simulink model "Function_Approximation_Ex1"  (R2024a)
settings: Solver=VariableStepAuto  StartTime=0.0  StopTime=512  RelTol=1e-3
undefined symbols (not defined in the file): S, vsva2197, xcvc1902
libraries: aieDSP x1, aieUtilities x1, vmcUtilities x1
settings Model: Creator=raghug  LastModifiedBy=sdegala
settings ConfigComp: CovBoundaryAbsTol=1.0e-5

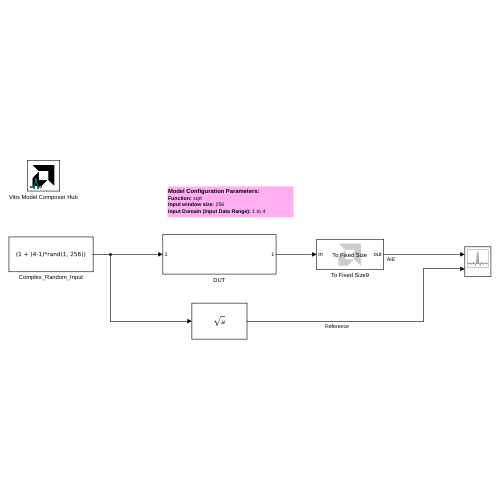
[thumbnail: Simulink's stored preview of the top-level diagram]
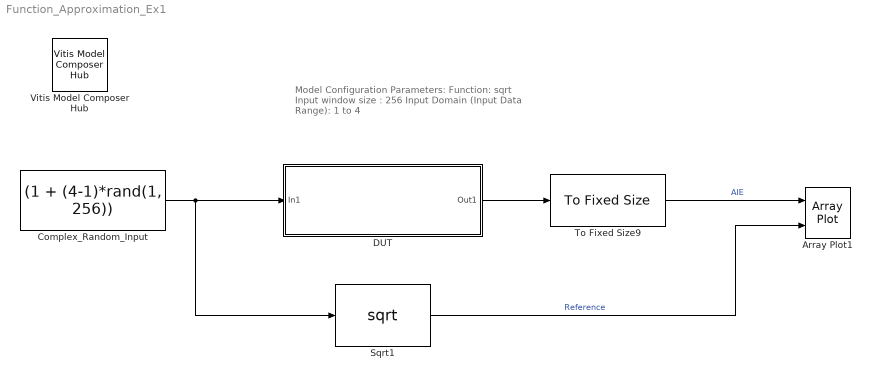
== system Function_Approximation_Ex1 ==
  note: Model Configuration Parameters:
      | Function: sqrt
      | Input window size : 256
      | Input Domain (Input Data Range): 1 to 4
  Array Plot1 : ArrayPlot  NumInputPorts=2  WindowPosition=[863.000000,486.000000,800.000000,500.000000,]  Visible=on  ScopeFrameLocation=window  YLimits=[0.8802 2.1161]  ShowLegend=on
  Complex_Random_Input : Constant  Value=(1 + (4-1)*rand(1, 256))  OutDataTypeStr=single  SampleTime=1
  DUT : Subsystem
  Sqrt1 : Sqrt
  To Fixed Size9 : aieUtilities/To Fixed Size  Mode=Stop simulation when input variable-size signal is not full  OutputSize=Inherit: Same as input  CopyMethod=Buffer samples to form output  HasStatusOutput=on
  Vitis Model Composer Hub : vmcUtilities/Vitis Model Composer Hub  Tag=genX  CodeGeneration=off  StartColumn=1  NumberOfColumns=1  TargetDirectory=./code  exportDesign=off  analyzeDesign=off  validateDesignOnHw=off  ExportType=AI Engines  IpVendor=xilinx.com  IpLibrary=hls  IpVersion=1.0  IpHWLanguage=Verilog  AieCompilerOptions={}  AieSimulatorOptions={}  CreateTestbench=off  TestbenchStackSize=10  RunRtlSim=off  RunCSim=off  RunAieSim=off  AieSimTimeout=50000  RunAieSimProfiling=off  LaunchVitisAnalyzer=off  PlotOutput=off  RunX86Sim=off  X86SimTimeout=10  GenHwImage=off  GenLibadfXo=off  GenHwValidationCode=off  PlatformType=Not Specified  HwSystemType=Baremetal  HwValidationTarget=hw  ProjDevice=xcvc1902-vsva2197-1LP-e-S  ProjDevicePart=xcvc1902-vsva2197-1LP-e-S  AIEType=AIE  SamplePeriod=-1  ClockFrequency=200  DataPathParallelism=1  xilinxfamily=versalaicore  part=xcvc1902  speed=-1LP-e-S  package=vsva2197  directory=./netlist  testbench=off  incr_netlist=off  synthesis_tool=Vivado  clock_wrapper=Clock Enables  dbl_ovrd=According to Block Masks  dcm_input_clock_period=10  sysclk_period=10  simulink_period=1  eval_field=0  LogFileName=''  NThreads=4
  wires:
  Complex_Random_Input/1 -> DUT/1(In1), Sqrt1/1
  To Fixed Size9/1 -> Array Plot1/1  "AIE"
  Sqrt1/1 -> Array Plot1/2  "Reference"
  DUT/1(Out1) -> To Fixed Size9/1

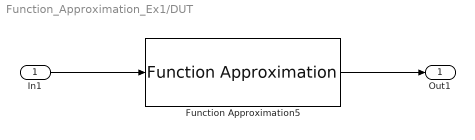
== system Function_Approximation_Ex1/DUT ==
  In1 : Inport
  Function Approximation5 : aieDSP/Function Approximation  AIE_VARIANT=1  data_type=float  coarse_bits=8  fine_bits=7  domain_mode=1 to 4 (2)  num_frames=256  shift_output=0  rnd_mode=Floor  sat_mode=Saturate  use_lut_reload=off  lookup_values=sqrt  blockJsonConstraints=[]  blockJsonConstraintsInternal=[]  spec=vmc_func_approx.json  SerializedMaskParamNames=[]  SerializedMaskParamValues=[]  SerializedMaskParamVisibilities=[]  block_type=Function Approximation  SerializedMaskParamDataypes=uint|typename|uint|uint|uint|uint|uint|uint|uint|uint|data_type  SerializedMaskParamEnumStrArr=0|0|0|0|0 to 1 (0),1 to 2 (1),1 to 4 (2)|0|0|Floor,Ceiling,Round to positive infinity,Round to negative infinity,Round symmetrical to infinity,Round symmetrical to zero,Round convergent to even,Round convergent to odd|None,Saturate,Symmetric|0|0  SerializedMaskParamEnumValArr=0|0|0|0|0,1,2|0|0|0,1,2,3,4,5,6,7|0,1,3|0|0  SerializedMaskParamVectorArr=0|0|0|0|0|0|0|0|0|0|1  SerializedMaskParamKeys=AIE_VARIANT|TT_DATA|TP_COARSE_BITS|TP_FINE_BITS|TP_DOMAIN_MODE|TP_WINDOW_VSIZE|TP_SHIFT|TP_RND|TP_SAT|TP_USE_LUT_RELOAD|lookup_values
  Out1 : Outport
  wires:
  In1/1 -> Function Approximation5/1
  Function Approximation5/1 -> Out1/1
